simulink model "MOIsolatedBuck3"  (R2013a)
settings: Solver=ode45  StartTime=0.0  StopTime=0.02  RelTol=1e-3
libraries: powerlib x18
settings Model: Creator=Sony  LastModifiedBy=Yooshaa

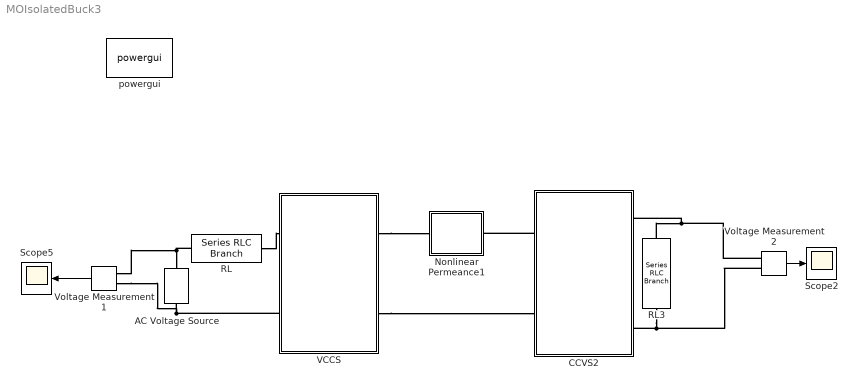
== system MOIsolatedBuck3 ==
  AC Voltage Source : powerlib/Electrical Sources/AC Voltage Source  Amplitude=200  Phase=0  Frequency=150e3  SampleTime=0  Measurements=None
  CCVS2 : Subsystem  mask{N=22}
  Nonlinear Permeance1 : Subsystem  mask{R=1e9, C=1e-5}
  RL : powerlib/Elements/Series RLC Branch  LConnTagsString=__new0  RConnTagsString=__new0  BranchType=RL  Resistance=1  Inductance=1e-5  SetiL0=off  InitialCurrent=0  Capacitance=1e-6  Setx0=off  InitialVoltage=0  Measurements=None
  RL3 : powerlib/Elements/Series RLC Branch  LConnTagsString=__new0  RConnTagsString=__new0  BranchType=R  Resistance=1  Inductance=1e-3  SetiL0=off  InitialCurrent=0  Capacitance=1e-6  Setx0=off  InitialVoltage=0  Measurements=None
  Scope2 : Scope
      settings: YMin=-600  YMax=600  SaveName=Vout
  Scope5 : Scope
      settings: YMin=-500  YMax=500  SaveName=Vin
  VCCS : Subsystem  mask{N=22}
  Voltage Measurement1 : powerlib/Measurements/Voltage Measurement  PhasorSimulation=off  OutputType=Complex  PSBequivalent=0
  Voltage Measurement2 : powerlib/Measurements/Voltage Measurement  PhasorSimulation=off  OutputType=Complex  PSBequivalent=0
  powergui : powerlib/powergui  Priority=1  SimulationMode=Discrete  SolverType=Backward Euler  SampleTime=1e-7  frequency=60  SPID=on  DisableSnubberDevices=off  DisableRonSwitches=off  DisableVfSwitches=off  SwTol=0  Interpol=off  DisplayEquations=off  frequencyindice=0  Pbase=100e6  ErrMax=1e-4  Iterations=50  UnitsV=kV  UnitsW=MW  FunctionMessages=off  echomessages=off  HookPort=off  EnableUseOfTLC=off  x0status=blocks  RestoreLinks=warning  ResistiveCurrentMeasurement=off  Frange=[0:2:500]  Ylog=off  Xlog=on  ShowGrid=off  save=off  variable=ZData  ZoomFFT=off  StartTime=0.0  cycles=1  DisplayStyle=1  fundamental=60  FreqAxis=off  MaxFrequency=1000  frequencyindicesteady=1  RmsSteady=1  display=off  Ts=0  methode=off
  wires:
  Voltage Measurement2/1 -> Scope2/1
  Voltage Measurement1/1 -> Scope5/1
  connections:
  RL/LConn1 -- Voltage Measurement1/LConn1 -- AC Voltage Source/RConn1
  VCCS/LConn2 -- AC Voltage Source/LConn1 -- Voltage Measurement1/LConn2
  VCCS/RConn1 -- Nonlinear Permeance1/LConn1
  RL/RConn1 -- VCCS/LConn1
  CCVS2/LConn1 -- Nonlinear Permeance1/RConn1
  VCCS/RConn2 -- CCVS2/LConn2
  Voltage Measurement2/LConn1 -- CCVS2/RConn1 -- RL3/RConn1
  Voltage Measurement2/LConn2 -- RL3/LConn1 -- CCVS2/RConn3

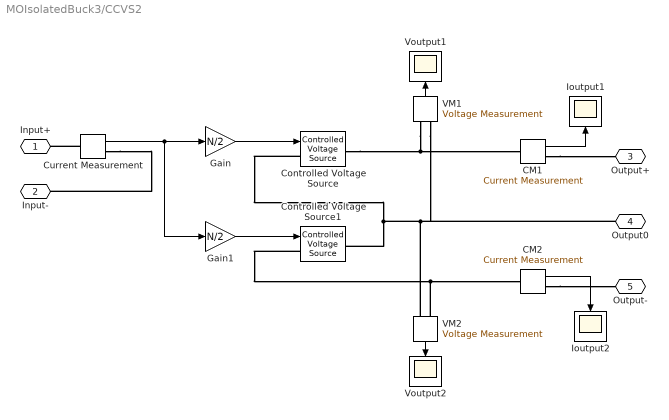
== system MOIsolatedBuck3/CCVS2 ==
  CM1 : powerlib/Measurements/Current Measurement  PhasorSimulation=off  OutputType=Complex  PSBequivalent=0
  CM2 : powerlib/Measurements/Current Measurement  PhasorSimulation=off  OutputType=Complex  PSBequivalent=0
  Controlled Voltage Source : powerlib/Electrical Sources/Controlled Voltage Source  Initialize=on  Source_Type=AC  Amplitude=0  Phase=0  Frequency=0  Measurements=None
  Controlled Voltage Source1 : powerlib/Electrical Sources/Controlled Voltage Source  Initialize=on  Source_Type=AC  Amplitude=0  Phase=0  Frequency=0  Measurements=None
  Current Measurement : powerlib/Measurements/Current Measurement  PhasorSimulation=off  OutputType=Complex  PSBequivalent=0
  Gain : Gain  Gain=N/2
  Gain1 : Gain  Gain=N/2
  Ioutput1 : Scope
      settings: YMin=-25  YMax=150  SaveName=Ioup
  Ioutput2 : Scope
      settings: YMin=-10  YMax=150  SaveName=Ioun
  VM1 : powerlib/Measurements/Voltage Measurement  PhasorSimulation=off  OutputType=Complex  PSBequivalent=0
  VM2 : powerlib/Measurements/Voltage Measurement  PhasorSimulation=off  OutputType=Complex  PSBequivalent=0
  Voutput1 : Scope
      settings: YMin=-20  YMax=20  SaveName=Voup
  Voutput2 : Scope
      settings: YMin=-20  YMax=20  SaveName=Voun
  Input+ : PMIOPort  Port=1  Side=Left
  Input- : PMIOPort  Port=2  Side=Left
  Output+ : PMIOPort  Port=3  Side=Right
  Output0 : PMIOPort  Port=4  Side=Right
  Output- : PMIOPort  Port=5  Side=Right
  wires:
  Gain/1 -> Controlled Voltage Source/1
  Current Measurement/1 -> Gain1/1, Gain/1
  Gain1/1 -> Controlled Voltage Source1/1
  VM2/1 -> Voutput2/1
  VM1/1 -> Voutput1/1
  CM2/1 -> Ioutput2/1
  CM1/1 -> Ioutput1/1
  connections:
  Current Measurement/LConn1 -- Input+/RConn1
  Current Measurement/RConn1 -- Input-/RConn1
  Controlled Voltage Source/RConn1 -- CM1/LConn1 -- VM1/LConn1
  Controlled Voltage Source/LConn1 -- Output0/RConn1 -- VM1/LConn2 -- VM2/LConn1 -- Controlled Voltage Source1/RConn1
  Controlled Voltage Source1/LConn1 -- VM2/LConn2 -- CM2/LConn1
  CM1/RConn1 -- Output+/RConn1
  CM2/RConn1 -- Output-/RConn1

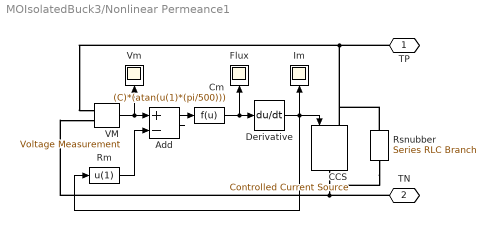
== system MOIsolatedBuck3/Nonlinear Permeance1 ==
  Add : Sum  Inputs=+-
  CCS : powerlib/Electrical Sources/Controlled Current Source  Initialize=on  Source_Type=AC  Amplitude=0  Phase=0  Frequency=0  Measurements=None
  Cm : Fcn  Expr=(C)*(atan(u(1)*(pi/500)))
  Derivative : Derivative
  Flux : Scope
      settings: YMin=-4e-05  YMax=4e-05  SaveName=PermeanceFlux
  Im : Scope
      settings: TimeRange=0.02  YMin=-200  YMax=200  SaveName=PermeanceIm
  Rm : Fcn  Expr=u(1)
  Rsnubber : powerlib/Elements/Series RLC Branch  LConnTagsString=__new0  RConnTagsString=__new0  BranchType=R  Resistance=R  Inductance=1e-3  SetiL0=off  InitialCurrent=0  Capacitance=1e-6  Setx0=off  InitialVoltage=0  Measurements=None
  VM : powerlib/Measurements/Voltage Measurement  PhasorSimulation=off  OutputType=Complex  PSBequivalent=0
  Vm : Scope
      settings: YMin=-4000  YMax=4000  SaveName=PermeanceVm
  TP : PMIOPort  Port=1  Side=Left
  TN : PMIOPort  Port=2  Side=Right
  wires:
  VM/1 -> Add/1, Vm/1
  Cm/1 -> Flux/1, Derivative/1
  Rm/1 -> Add/2
  Derivative/1 -> Rm/1, CCS/1, Im/1
  Add/1 -> Cm/1
  connections:
  TN/RConn1 -- Rsnubber/RConn1 -- CCS/RConn1 -- VM/LConn2
  TP/RConn1 -- Rsnubber/LConn1 -- CCS/LConn1 -- VM/LConn1

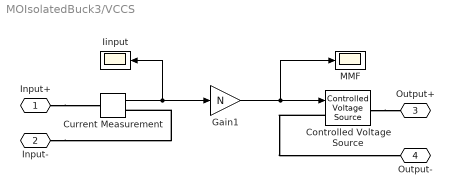
== system MOIsolatedBuck3/VCCS ==
  Controlled Voltage Source : powerlib/Electrical Sources/Controlled Voltage Source  Initialize=off  Source_Type=AC  Amplitude=0  Phase=0  Frequency=0  Measurements=None
  Current Measurement : powerlib/Measurements/Current Measurement  PhasorSimulation=off  OutputType=Complex  PSBequivalent=0
  Gain1 : Gain  Gain=N
  Iinput : Scope
      settings: YMin=-100  YMax=100  SaveName=Iprimary
  MMF : Scope
      settings: YMin=-11000  YMax=11000  SaveName=MMF
  Input+ : PMIOPort  Port=1  Side=Left
  Input- : PMIOPort  Port=2  Side=Left
  Output+ : PMIOPort  Port=3  Side=Right
  Output- : PMIOPort  Port=4  Side=Right
  wires:
  Current Measurement/1 -> Iinput/1, Gain1/1
  Gain1/1 -> MMF/1, Controlled Voltage Source/1
  connections:
  Input+/RConn1 -- Current Measurement/LConn1
  Input-/RConn1 -- Current Measurement/RConn1
  Controlled Voltage Source/RConn1 -- Output+/RConn1
  Controlled Voltage Source/LConn1 -- Output-/RConn1
